simulink model "ControlePD_ind2015"  (R2015a)
settings: Solver=ode3  SolverMode=SingleTasking  StartTime=0.0  StopTime=10.0  FixedStep=Ts
values from neighbouring files (symbols this model uses):
  Beff = 50    [Ex4.m]
  Jeff = 2.2    [Ex4.m]
  K = 17.7    [Ex4.m]
  Kd = (2*qsi*wn*Jeff - Beff)/K    (= -0.338983050847)    [Ex4.m]
  Kp = (wn^2*Jeff)/K    (= 12.4293785311)    [Ex4.m]
  N = 10    [Ex4.m]
  r = 1    [Ex4.m]
  SP_theta = [60;-110;20;20;20]    [Ex4.m]
(part 1 of 3)
settings Model: CovMetricSettings=dwe  CovHtmlReporting=off  covSaveCumulativeToWorkspaceVar=off  CovSaveSingleToWorkspaceVar=off  CovExternalEMLEnable=on  Creator=Karoline  LastModifiedBy=lunet
settings DataIOCC: LimitDataPoints=off  SaveFormat=Dataset
settings DebuggingCC: SFUnexpectedBacktrackingDiag=error  SFNoUnconditionalDefaultTransitionDiag=error
settings HardwareCC: ProdBitPerPointer=64  ProdLargestAtomicFloat=Float  ProdIntDivRoundTo=Zero  ProdEndianess=LittleEndian  ProdHWDeviceType=Specified
settings ModelReferenceCC: PropagateSignalLabelsOutOfModel=on
settings GRTTargetCC: TargetLangStandard=C99 (ISO)

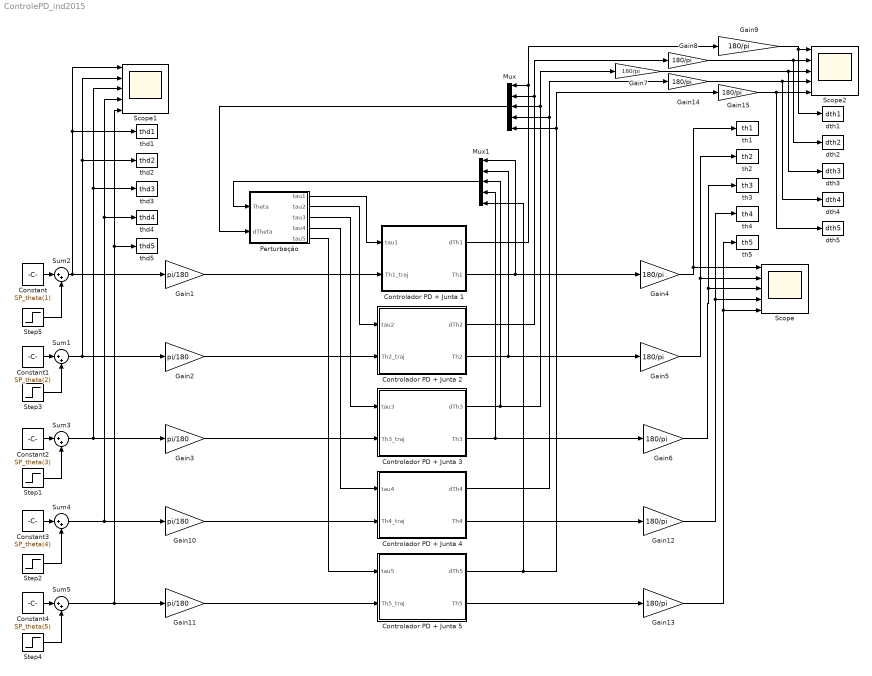
== system ControlePD_ind2015 ==
  Constant : Constant  Value=SP_theta(1)
  Constant1 : Constant  Value=SP_theta(2)
  Constant2 : Constant  Value=SP_theta(3)
  Constant3 : Constant  Value=SP_theta(4)
  Constant4 : Constant  Value=SP_theta(5)
  Controlador PD + Junta 1 : Subsystem
  Controlador PD + Junta 2 : Subsystem
  Controlador PD + Junta 3 : Subsystem
  Controlador PD + Junta 4 : Subsystem
  Controlador PD + Junta 5 : Subsystem
  Gain{1..3,10..11} (5 alike) : Gain  Gain=pi/180
  Gain{4..9,12..15} (10 alike) : Gain  Gain=180/pi
  Mux : Mux  Inputs=5
  Mux1 : Mux  Inputs=5
  Perturbação : Subsystem
  Scope : Scope  NumInputPorts=5
      settings: TimeRange=auto  MaxDataPoints=5000  SaveToWorkspace=off  SaveName=ScopeData  YMin=-133.87767~-5~-5~-5~-5  YMax=81.54196~5~5~5~5  SampleTime=-1
  Scope1 : Scope  NumInputPorts=5
      settings: TimeRange=auto  MaxDataPoints=5000  SaveToWorkspace=off  YMin=-131.25~-5~-5~-5~-5  YMax=81.25~5~5~5~5  SampleTime=-1
  Scope2 : Scope  NumInputPorts=5
      settings: TimeRange=auto  MaxDataPoints=5000  SaveToWorkspace=off  SaveName=ScopeData5  YMin=-33.93434~-5~-5~-5~-5  YMax=205.40908~5~5~5~5  SampleTime=-1
  Step{1..2,4..5} (4 alike) : Step  Time=0  After=0  SampleTime=0
  Step3 : Step  Time=3  After=60  SampleTime=0
  Sum{1..5} (5 alike) : Sum  Inputs=|++
  dth1 : ToWorkspace  VariableName=dth1  SampleTime=-1
  dth2 : ToWorkspace  VariableName=dth2  SampleTime=-1
  dth3 : ToWorkspace  VariableName=dth3  SampleTime=-1
  dth4 : ToWorkspace  VariableName=dth4  SampleTime=-1
  dth5 : ToWorkspace  VariableName=dth5  SampleTime=-1
  th1 : ToWorkspace  VariableName=th1  SampleTime=-1
  th2 : ToWorkspace  VariableName=th2  SampleTime=-1
  th3 : ToWorkspace  VariableName=th3  SampleTime=-1
  th4 : ToWorkspace  VariableName=th4  SampleTime=-1
  th5 : ToWorkspace  VariableName=th5  SampleTime=-1
  "thd1 " : ToWorkspace  VariableName=thd1  SampleTime=-1
  "thd2 " : ToWorkspace  VariableName=thd2  SampleTime=-1
  thd3 : ToWorkspace  VariableName=thd3  SampleTime=-1
  thd4 : ToWorkspace  VariableName=thd4  SampleTime=-1
  thd5 : ToWorkspace  VariableName=thd5  SampleTime=-1
  wires:
  Perturbação/1(tau1) -> Controlador PD + Junta 1/1(tau1)
  Mux/1 -> Perturbação/2(dTheta)
  Mux1/1 -> Perturbação/1(Theta)
  Step3/1 -> Sum1/2
  Sum1/1 -> Scope1/2, "thd2 "/1, Gain2/1
  Constant1/1 -> Sum1/1
  Gain1/1 -> Controlador PD + Junta 1/2(Th1_traj)
  Gain2/1 -> Controlador PD + Junta 2/2(Th2_traj)
  Gain3/1 -> Controlador PD + Junta 3/2(Th3_traj)
  Gain4/1 -> th1/1, Scope/1
  Gain5/1 -> th2/1, Scope/2
  Gain6/1 -> th3/1, Scope/3
  Controlador PD + Junta 1/1("dTh1 ") -> Mux/1, Gain9/1
  Controlador PD + Junta 2/1("dTh2 ") -> Mux/2, Gain8/1
  Controlador PD + Junta 3/1("dTh3 ") -> Mux1/3, Mux/3, Gain7/1
  Controlador PD + Junta 1/2(Th1) -> Mux1/1, Gain4/1
  Controlador PD + Junta 2/2(Th2) -> Mux1/2, Gain5/1
  Controlador PD + Junta 3/2(Th3) -> Mux1/4, Gain6/1
  Perturbação/2(tau2) -> Controlador PD + Junta 2/1(tau2)
  Perturbação/3(tau3) -> Controlador PD + Junta 3/1(tau3)
  Gain7/1 -> dth3/1, Scope2/3
  Gain8/1 -> dth2/1, Scope2/2
  Gain9/1 -> dth1/1, Scope2/1
  Gain10/1 -> Controlador PD + Junta 4/2(Th4_traj)
  Gain11/1 -> Controlador PD + Junta 5/2(Th5_traj)
  Constant/1 -> Sum2/1
  Constant2/1 -> Sum3/1
  Constant3/1 -> Sum4/1
  Constant4/1 -> Sum5/1
  Step1/1 -> Sum3/2
  Step2/1 -> Sum4/2
  Step4/1 -> Sum5/2
  Sum5/1 -> thd5/1, Scope1/5, Gain11/1
  Sum3/1 -> Gain3/1, Scope1/3, thd3/1
  Step5/1 -> Sum2/2
  Sum2/1 -> Scope1/1, "thd1 "/1, Gain1/1
  Sum4/1 -> thd4/1, Scope1/4, Gain10/1
  Controlador PD + Junta 4/2(Th4) -> Gain12/1
  Controlador PD + Junta 5/2(Th5) -> Gain13/1
  Gain12/1 -> Scope/4, th4/1
  Gain13/1 -> Scope/5, th5/1
  Gain14/1 -> dth4/1, Scope2/4
  Controlador PD + Junta 4/1("dTh4 ") -> Mux/4, Gain14/1
  Gain15/1 -> dth5/1, Scope2/5
  Controlador PD + Junta 5/1("dTh5 ") -> Mux1/5, Mux/5, Gain15/1
  Perturbação/4(tau4) -> Controlador PD + Junta 4/1(tau4)
  Perturbação/5(tau5) -> Controlador PD + Junta 5/1(tau5)

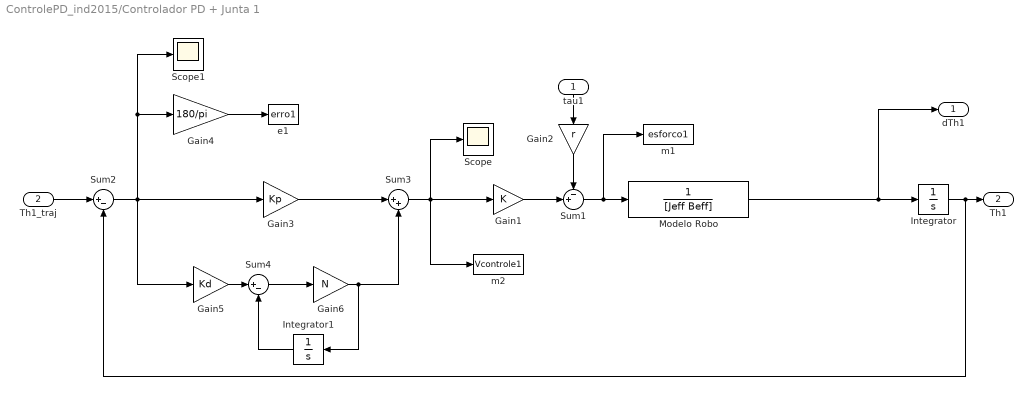
== system ControlePD_ind2015/Controlador PD + Junta 1 ==
  tau1 : Inport
  Th1_traj : Inport  Port=2
  Gain1 : Gain  Gain=K
  Gain2 : Gain  Gain=r
  Gain3 : Gain  Gain=Kp
  Gain4 : Gain  Gain=180/pi
  Gain5 : Gain  Gain=Kd
  Gain6 : Gain  Gain=N
  Integrator : Integrator  InitialCondition=SP_theta(1)*pi/180
  Integrator1 : Integrator
  Modelo Robo : TransferFcn  Denominator=[Jeff Beff]
  Scope : Scope
      settings: TimeRange=auto  MaxDataPoints=5000  SaveToWorkspace=off  YMin=-4.89691  YMax=11.84583  SampleTime=-1
  Scope1 : Scope
      settings: TimeRange=auto  MaxDataPoints=5000  SaveToWorkspace=off  SaveName=ScopeData6  YMin=-0.42473  YMax=1.21038  SampleTime=-1
  Sum1 : Sum  Inputs=-+|
  Sum2 : Sum  Inputs=|+-
  Sum3 : Sum  Inputs=|++
  Sum4 : Sum  Inputs=|+-
  e1 : ToWorkspace  VariableName=erro1  SampleTime=-1
  m1 : ToWorkspace  VariableName=esforco1  SampleTime=-1
  m2 : ToWorkspace  VariableName=Vcontrole1  SampleTime=-1
  "dTh1 " : Outport
  Th1 : Outport  Port=2
  wires:
  tau1/1 -> Gain2/1
  Gain1/1 -> Sum1/2
  Sum1/1 -> m1/1, Modelo Robo/1
  Integrator/1 -> Th1/1, Sum2/2
  Th1_traj/1 -> Sum2/1
  Gain2/1 -> Sum1/1
  Sum2/1 -> Gain5/1, Gain3/1, Scope1/1, Gain4/1
  Gain4/1 -> e1/1
  Gain3/1 -> Sum3/1
  Gain5/1 -> Sum4/1
  Sum4/1 -> Gain6/1
  Gain6/1 -> Sum3/2, Integrator1/1
  Integrator1/1 -> Sum4/2
  Sum3/1 -> m2/1, Scope/1, Gain1/1
  Modelo Robo/1 -> "dTh1 "/1, Integrator/1

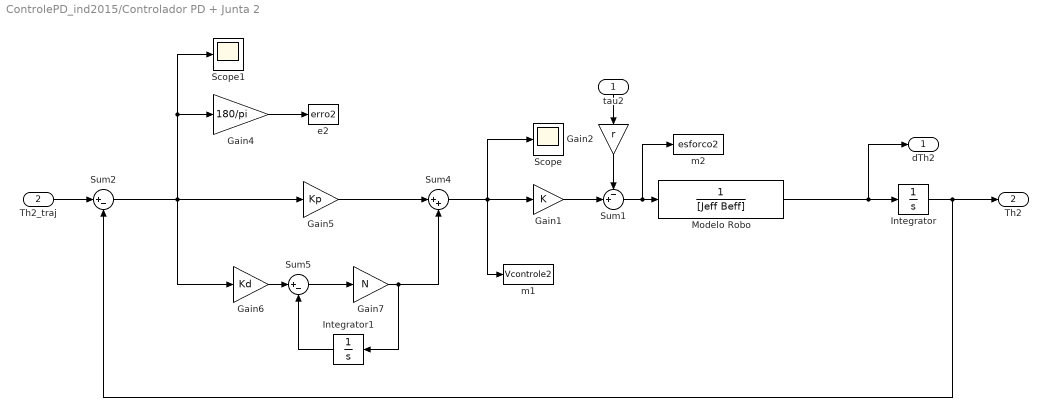
== system ControlePD_ind2015/Controlador PD + Junta 2 ==
  tau2 : Inport
  Th2_traj : Inport  Port=2
  Gain1 : Gain  Gain=K
  Gain2 : Gain  Gain=r
  Gain4 : Gain  Gain=180/pi
  Gain5 : Gain  Gain=Kp
  Gain6 : Gain  Gain=Kd
  Gain7 : Gain  Gain=N
  Integrator : Integrator  InitialCondition=SP_theta(2)*pi/180
  Integrator1 : Integrator
  "Modelo Robo " : TransferFcn  Denominator=[Jeff Beff]
  Scope : Scope
      settings: TimeRange=auto  MaxDataPoints=5000  SaveToWorkspace=off  SaveName=ScopeData2  YMin=-10  YMax=10  SampleTime=-1
  Scope1 : Scope
      settings: TimeRange=auto  MaxDataPoints=5000  SaveToWorkspace=off  SaveName=ScopeData5  YMin=-10  YMax=10  SampleTime=-1
  Sum1 : Sum  Inputs=-+|
  Sum2 : Sum  Inputs=|+-
  Sum4 : Sum  Inputs=|++
  Sum5 : Sum  Inputs=|+-
  e2 : ToWorkspace  VariableName=erro2  SampleTime=-1
  m1 : ToWorkspace  VariableName=Vcontrole2  SampleTime=-1
  m2 : ToWorkspace  VariableName=esforco2  SampleTime=-1
  "dTh2 " : Outport
  Th2 : Outport  Port=2
  wires:
  tau2/1 -> Gain2/1
  Gain1/1 -> Sum1/2
  Sum1/1 -> m2/1, "Modelo Robo "/1
  Integrator/1 -> Th2/1, Sum2/2
  Th2_traj/1 -> Sum2/1
  Gain2/1 -> Sum1/1
  Gain4/1 -> e2/1
  Gain5/1 -> Sum4/1
  Sum2/1 -> Scope1/1, Gain4/1, Gain6/1, Gain5/1
  Integrator1/1 -> Sum5/2
  Sum5/1 -> Gain7/1
  Gain6/1 -> Sum5/1
  Gain7/1 -> Sum4/2, Integrator1/1
  Sum4/1 -> m1/1, Scope/1, Gain1/1
  "Modelo Robo "/1 -> "dTh2 "/1, Integrator/1

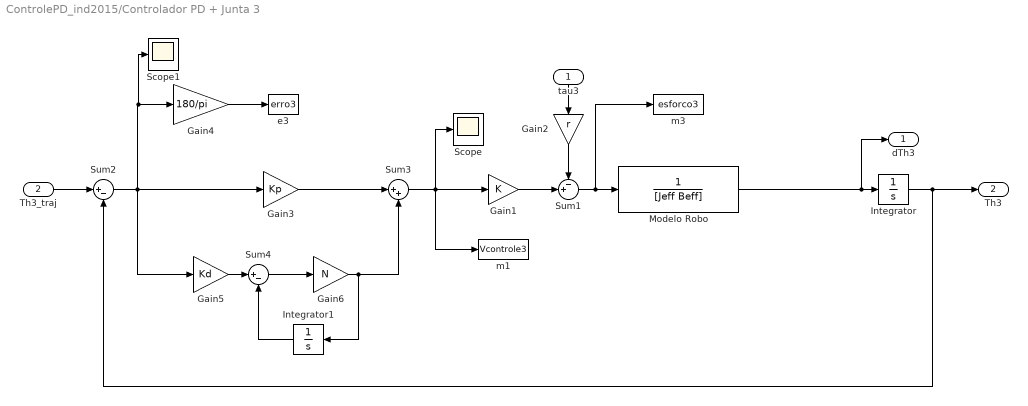
== system ControlePD_ind2015/Controlador PD + Junta 3 ==
  tau3 : Inport
  Th3_traj : Inport  Port=2
  Gain1 : Gain  Gain=K
  Gain2 : Gain  Gain=r
  Gain3 : Gain  Gain=Kp
  Gain4 : Gain  Gain=180/pi
  Gain5 : Gain  Gain=Kd
  Gain6 : Gain  Gain=N
  Integrator : Integrator  InitialCondition=SP_theta(3)*pi/180
  Integrator1 : Integrator
  Modelo Robo : TransferFcn  Denominator=[Jeff Beff]
  Scope : Scope
      settings: TimeRange=auto  MaxDataPoints=5000  SaveToWorkspace=off  SaveName=ScopeData3  YMin=-10  YMax=10  SampleTime=-1
  Scope1 : Scope
      settings: TimeRange=auto  MaxDataPoints=5000  SaveToWorkspace=off  SaveName=ScopeData4  YMin=-10  YMax=10  SampleTime=-1
  Sum1 : Sum  Inputs=-+|
  Sum2 : Sum  Inputs=|+-
  Sum3 : Sum  Inputs=|++
  Sum4 : Sum  Inputs=|+-
  e3 : ToWorkspace  VariableName=erro3  SampleTime=-1
  m1 : ToWorkspace  VariableName=Vcontrole3  SampleTime=-1
  m3 : ToWorkspace  VariableName=esforco3  SampleTime=-1
  "dTh3 " : Outport
  Th3 : Outport  Port=2
  wires:
  tau3/1 -> Gain2/1
  Gain1/1 -> Sum1/2
  Sum1/1 -> m3/1, Modelo Robo/1
  Integrator/1 -> Th3/1, Sum2/2
  Th3_traj/1 -> Sum2/1
  Gain2/1 -> Sum1/1
  Gain4/1 -> e3/1
  Gain3/1 -> Sum3/1
  Sum2/1 -> Scope1/1, Gain4/1, Gain5/1, Gain3/1
  Integrator1/1 -> Sum4/2
  Sum4/1 -> Gain6/1
  Gain5/1 -> Sum4/1
  Gain6/1 -> Sum3/2, Integrator1/1
  Sum3/1 -> m1/1, Scope/1, Gain1/1
  Modelo Robo/1 -> Integrator/1, "dTh3 "/1

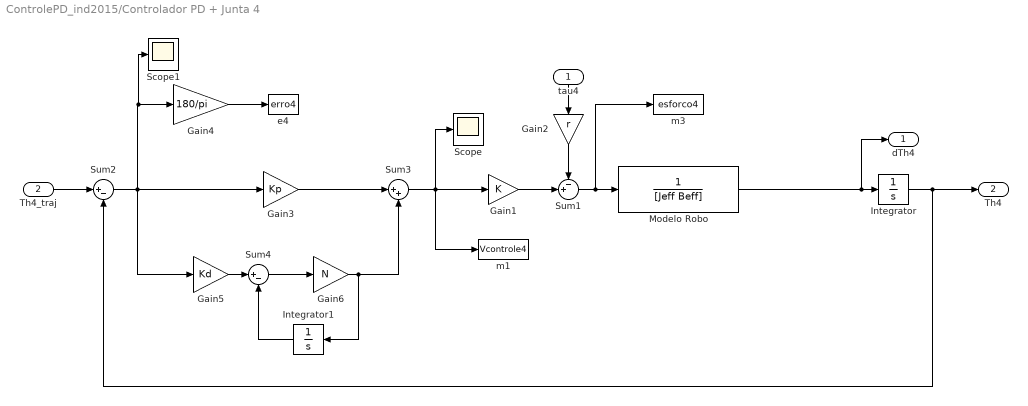
== system ControlePD_ind2015/Controlador PD + Junta 4 ==
  tau4 : Inport
  Th4_traj : Inport  Port=2
  Gain1 : Gain  Gain=K
  Gain2 : Gain  Gain=r
  Gain3 : Gain  Gain=Kp
  Gain4 : Gain  Gain=180/pi
  Gain5 : Gain  Gain=Kd
  Gain6 : Gain  Gain=N
  Integrator : Integrator  InitialCondition=SP_theta(4)*pi/180
  Integrator1 : Integrator
  Modelo Robo : TransferFcn  Denominator=[Jeff Beff]
  Scope : Scope
      settings: TimeRange=auto  MaxDataPoints=5000  SaveToWorkspace=off  SaveName=ScopeData3  YMin=-10  YMax=10  SampleTime=-1
  Scope1 : Scope
      settings: TimeRange=auto  MaxDataPoints=5000  SaveToWorkspace=off  SaveName=ScopeData4  YMin=-10  YMax=10  SampleTime=-1
  Sum1 : Sum  Inputs=-+|
  Sum2 : Sum  Inputs=|+-
  Sum3 : Sum  Inputs=|++
  Sum4 : Sum  Inputs=|+-
  e4 : ToWorkspace  VariableName=erro4  SampleTime=-1
  m1 : ToWorkspace  VariableName=Vcontrole4  SampleTime=-1
  m3 : ToWorkspace  VariableName=esforco4  SampleTime=-1
  "dTh4 " : Outport
  Th4 : Outport  Port=2
  wires:
  tau4/1 -> Gain2/1
  Gain1/1 -> Sum1/2
  Sum1/1 -> m3/1, Modelo Robo/1
  Integrator/1 -> Th4/1, Sum2/2
  Th4_traj/1 -> Sum2/1
  Gain2/1 -> Sum1/1
  Gain4/1 -> e4/1
  Gain3/1 -> Sum3/1
  Sum2/1 -> Scope1/1, Gain4/1, Gain5/1, Gain3/1
  Integrator1/1 -> Sum4/2
  Sum4/1 -> Gain6/1
  Gain5/1 -> Sum4/1
  Gain6/1 -> Sum3/2, Integrator1/1
  Sum3/1 -> m1/1, Scope/1, Gain1/1
  Modelo Robo/1 -> Integrator/1, "dTh4 "/1

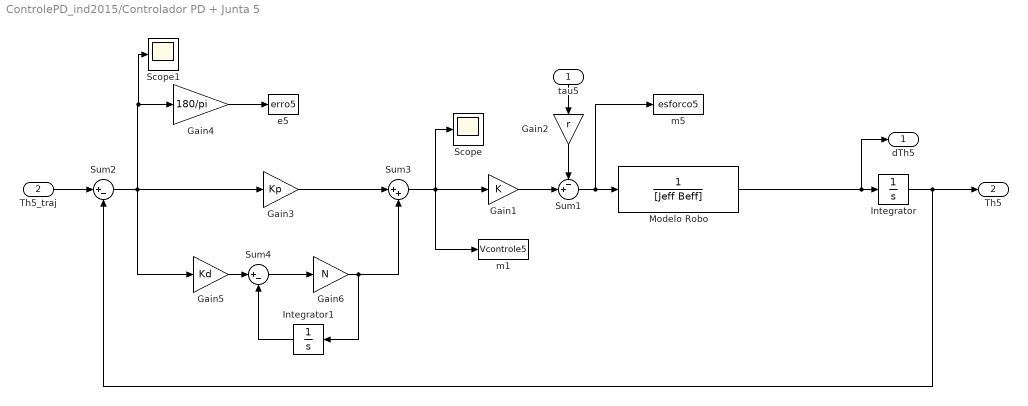
== system ControlePD_ind2015/Controlador PD + Junta 5 ==
  tau5 : Inport
  Th5_traj : Inport  Port=2
  Gain1 : Gain  Gain=K
  Gain2 : Gain  Gain=r
  Gain3 : Gain  Gain=Kp
  Gain4 : Gain  Gain=180/pi
  Gain5 : Gain  Gain=Kd
  Gain6 : Gain  Gain=N
  Integrator : Integrator  InitialCondition=SP_theta(5)*pi/180
  Integrator1 : Integrator
  Modelo Robo : TransferFcn  Denominator=[Jeff Beff]
  Scope : Scope
      settings: TimeRange=auto  MaxDataPoints=5000  SaveToWorkspace=off  SaveName=ScopeData3  YMin=-10  YMax=10  SampleTime=-1
  Scope1 : Scope
      settings: TimeRange=auto  MaxDataPoints=5000  SaveToWorkspace=off  SaveName=ScopeData4  YMin=-10  YMax=10  SampleTime=-1
  Sum1 : Sum  Inputs=-+|
  Sum2 : Sum  Inputs=|+-
  Sum3 : Sum  Inputs=|++
  Sum4 : Sum  Inputs=|+-
  e5 : ToWorkspace  VariableName=erro5  SampleTime=-1
  m1 : ToWorkspace  VariableName=Vcontrole5  SampleTime=-1
  m5 : ToWorkspace  VariableName=esforco5  SampleTime=-1
  "dTh5 " : Outport
  Th5 : Outport  Port=2
  wires:
  tau5/1 -> Gain2/1
  Gain1/1 -> Sum1/2
  Sum1/1 -> m5/1, Modelo Robo/1
  Integrator/1 -> Th5/1, Sum2/2
  Th5_traj/1 -> Sum2/1
  Gain2/1 -> Sum1/1
  Gain4/1 -> e5/1
  Gain3/1 -> Sum3/1
  Sum2/1 -> Scope1/1, Gain4/1, Gain5/1, Gain3/1
  Integrator1/1 -> Sum4/2
  Sum4/1 -> Gain6/1
  Gain5/1 -> Sum4/1
  Gain6/1 -> Sum3/2, Integrator1/1
  Sum3/1 -> m1/1, Scope/1, Gain1/1
  Modelo Robo/1 -> Integrator/1, "dTh5 "/1

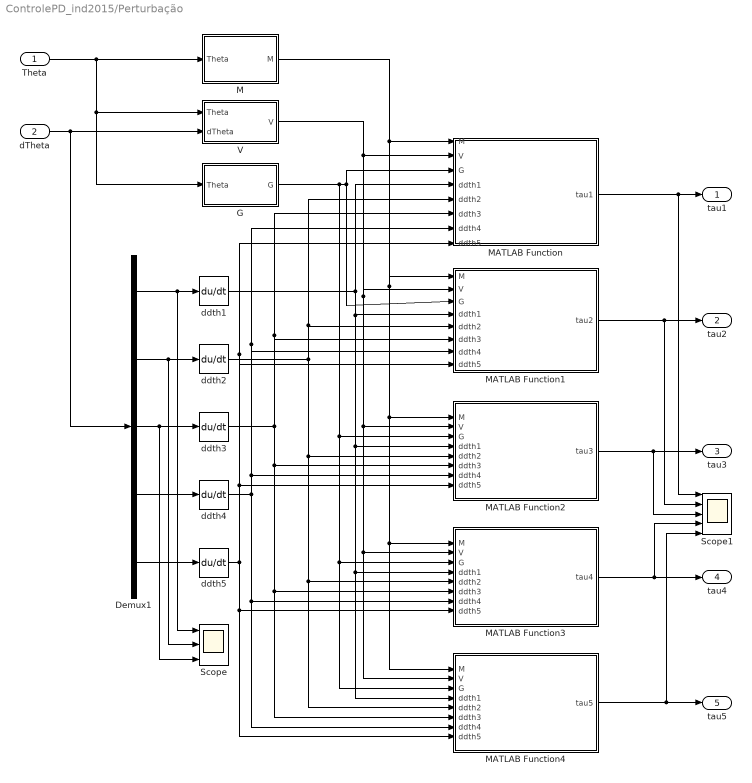
== system ControlePD_ind2015/Perturbação ==
  Theta : Inport
  dTheta : Inport  Port=2
  Demux1 : Demux  Outputs=5
  G : Subsystem
  M : Subsystem
  MATLAB Function : MATLAB Function  TreatAsAtomicUnit=on
      settings: PermitHierarchicalResolution=ParametersOnly
  MATLAB Function1 : MATLAB Function  TreatAsAtomicUnit=on
      settings: PermitHierarchicalResolution=ParametersOnly
  MATLAB Function2 : MATLAB Function  TreatAsAtomicUnit=on
      settings: PermitHierarchicalResolution=ParametersOnly
  MATLAB Function3 : MATLAB Function  TreatAsAtomicUnit=on
      settings: PermitHierarchicalResolution=ParametersOnly
  MATLAB Function4 : MATLAB Function  TreatAsAtomicUnit=on
      settings: PermitHierarchicalResolution=ParametersOnly
  Scope : Scope  NumInputPorts=3
      settings: TimeRange=auto  MaxDataPoints=5000  SaveToWorkspace=off  SaveName=ScopeData6  YMin=-10~-5~-5  YMax=10~5~5  SampleTime=-1
  Scope1 : Scope  NumInputPorts=5
      settings: TimeRange=auto  MaxDataPoints=5000  SaveToWorkspace=off  SaveName=ScopeData7  YMin=-10~-5~-5~-5~-5  YMax=10~5~5~5~5  SampleTime=-1
  V : Subsystem
  ddth{1..5} (5 alike) : Derivative
  tau1 : Outport
  tau2 : Outport  Port=2
  tau3 : Outport  Port=3
  tau4 : Outport  Port=4
  tau5 : Outport  Port=5
  wires:
  dTheta/1 -> Demux1/1, V/2(dTheta)
  G/1(G) -> MATLAB Function1/3(G), MATLAB Function/3(G), MATLAB Function4/3(G), MATLAB Function3/3(G), MATLAB Function2/3(G)
  V/1(V) -> MATLAB Function1/2(V), MATLAB Function4/2(V), MATLAB Function3/2(V), MATLAB Function2/2(V), MATLAB Function/2(V)
  Theta/1 -> M/1(Theta), G/1(Theta), V/1(Theta)
  Demux1/1 -> Scope/1, ddth1/1
  Demux1/2 -> Scope/2, ddth2/1
  Demux1/3 -> Scope/3, ddth3/1
  MATLAB Function/1(tau1) -> tau1/1, Scope1/1
  MATLAB Function1/1(tau2) -> tau2/1, Scope1/2
  MATLAB Function2/1(tau3) -> Scope1/3, tau3/1
  Demux1/4 -> ddth4/1
  Demux1/5 -> ddth5/1
  M/1(M) -> MATLAB Function4/1(M), MATLAB Function3/1(M), MATLAB Function2/1(M), MATLAB Function1/1(M), MATLAB Function/1(M)
  ddth1/1 -> MATLAB Function4/4(ddth1), MATLAB Function3/4(ddth1), MATLAB Function2/4(ddth1), MATLAB Function1/4(ddth1), MATLAB Function/4(ddth1)
  ddth2/1 -> MATLAB Function4/5(ddth2), MATLAB Function3/5(ddth2), MATLAB Function2/5(ddth2), MATLAB Function1/5(ddth2), MATLAB Function/5(ddth2)
  ddth3/1 -> MATLAB Function1/6(ddth3), MATLAB Function/6(ddth3), MATLAB Function4/6(ddth3), MATLAB Function3/6(ddth3), MATLAB Function2/6(ddth3)
  ddth4/1 -> MATLAB Function2/7(ddth4), MATLAB Function1/7(ddth4), MATLAB Function/7(ddth4), MATLAB Function4/7(ddth4), MATLAB Function3/7(ddth4)
  ddth5/1 -> MATLAB Function2/8(ddth5), MATLAB Function1/8(ddth5), MATLAB Function/8(ddth5), MATLAB Function4/8(ddth5), MATLAB Function3/8(ddth5)
  MATLAB Function3/1(tau4) -> Scope1/4, tau4/1
  MATLAB Function4/1(tau5) -> Scope1/5, tau5/1

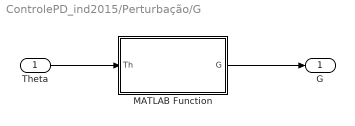
== system ControlePD_ind2015/Perturbação/G ==
  Theta : Inport
  MATLAB Function : MATLAB Function  TreatAsAtomicUnit=on
      settings: PermitHierarchicalResolution=ParametersOnly
  G : Outport
  wires:
  Theta/1 -> MATLAB Function/1(Th)
  MATLAB Function/1(G) -> G/1

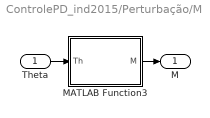
== system ControlePD_ind2015/Perturbação/M ==
  Theta : Inport
  MATLAB Function3 : MATLAB Function  TreatAsAtomicUnit=on
      settings: PermitHierarchicalResolution=ParametersOnly
  M : Outport
  wires:
  Theta/1 -> MATLAB Function3/1(Th)
  MATLAB Function3/1(M) -> M/1

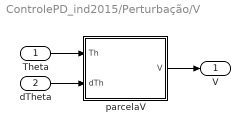
== system ControlePD_ind2015/Perturbação/V ==
  Theta : Inport
  dTheta : Inport  Port=2
  parcelaV : MATLAB Function  TreatAsAtomicUnit=on
      settings: PermitHierarchicalResolution=ParametersOnly
  V : Outport
  wires:
  parcelaV/1(V) -> V/1
  Theta/1 -> parcelaV/1(Th)
  dTheta/1 -> parcelaV/2(dTh)

== matlab function ControlePD_ind2015/Perturbação/MATLAB Function3 ==
  data: M input; V input; tau4 output; G input; ddth1 input; ddth2 input; ddth3 input; ddth4 input; ddth5 input
function tau4  = calcul_dk4(M, V, G,ddth1,ddth2,ddth3,ddth4,ddth5)

ddth = [ddth1; ddth2; ddth3; ddth4; ddth5];

tau4 = M(4,:)*ddth + V(4,1) + G(4);

== matlab function ControlePD_ind2015/Perturbação/G/MATLAB Function ==
  data: Th input; G output
function G = calcul_G(Th)

th1 = Th(1);
th2 = Th(2);
th3 = Th(3);
th4 = Th(4);
th5 = Th(5);
g = 9.81;

G = [                                                                                                                                                                                                                                                                                               0;
 -g*((49*cos(th2)*sin(th3))/125 - cos(th2)/2 + (49*cos(th3)*sin(th2))/125 + (3*cos(th2)*cos(th5)*sin(th3))/40 + (3*cos(th3)*cos(th5)*sin(th2))/40 + (3*cos(th2)*cos(th3)*cos(th4)*sin(th5))/40 - (3*cos(th4)*sin(th2)*sin(th3)*sin(th5))/40);
                 -g*((49*cos(th2)*sin(th3))/125 + (49*cos(th3)*sin(th2))/125 + (3*cos(th2)*cos(th5)*sin(th3))/40 + (3*cos(th3)*cos(th5)*sin(th2))/40 + (3*cos(th2)*cos(th3)*cos(th4)*sin(th5))/40 - (3*cos(th4)*sin(th2)*sin(th3)*sin(th5))/40);
                                                                                                                                                                                                                                                (3*g*sin(th4)*sin(th5)*sin(th2 + th3))/40;
                                                                                       -g*((3*cos(th2)*cos(th3)*sin(th5))/40 - (3*sin(th2)*sin(th3)*sin(th5))/40 + (3*cos(th2)*cos(th4)*cos(th5)*sin(th3))/40 + (3*cos(th3)*cos(th4)*cos(th5)*sin(th2))/40)];

== matlab function ControlePD_ind2015/Perturbação/MATLAB Function1 ==
  data: M input; V input; tau2 output; G input; ddth1 input; ddth2 input; ddth3 input; ddth4 input; ddth5 input
function tau2  = calcul_dk2(M,V,G,ddth1,ddth2,ddth3,ddth4,ddth5)

ddth = [ddth1; ddth2; ddth3; ddth4; ddth5];

tau2 = M(2,:)*ddth + V(2,1) + G(2);

== matlab function ControlePD_ind2015/Perturbação/MATLAB Function ==
  data: M input; V input; tau1 output; G input; ddth1 input; ddth2 input; ddth3 input; ddth4 input; ddth5 input
function tau1  = calcul_dk1(M,V,G,ddth1,ddth2,ddth3,ddth4,ddth5)

ddth = [ddth1; ddth2; ddth3; ddth4; ddth5];

tau1 = M(1,:)*ddth + V(1,1) + G(1);

== matlab function ControlePD_ind2015/Perturbação/MATLAB Function2 ==
  data: M input; V input; tau3 output; G input; ddth1 input; ddth2 input; ddth3 input; ddth4 input; ddth5 input
function tau3  = calcul_dk3(M, V, G,ddth1,ddth2,ddth3,ddth4,ddth5)

ddth = [ddth1; ddth2; ddth3; ddth4; ddth5];

tau3 = M(3,:)*ddth + V(3,1) + G(3);

== matlab function ControlePD_ind2015/Perturbação/M/MATLAB Function3 ==
  data: Th input; M output
function M = calcul_M(Th)

th1 = Th(1);
th2 = Th(2);
th3 = Th(3);
th4 = Th(4);
th5 = Th(5);

M = [ (87*cos(th2)^2*cos(th5))/2500 + (87*cos(th3)^2*cos(th5))/2500 - (33*cos(th2)^2*sin(th3))/50 + (53231*cos(th2)^2)/62500 + (8453*cos(th3)^2)/31250 - (9*cos(th5)^2)/3200 - (8453*cos(th2)^2*cos(th3)^2)/15625 - (217*cos(th2)^2*cos(th4)^2)/80000 + (9*cos(th2)^2*cos(th5)^2)/3200 - (217*cos(th3)^2*cos(th4)^2)/80000 + (9*cos(th3)^2*cos(th5)^2)/3200 - (87*cos(th2)^2*cos(th3)^2*cos(th5))/1250 - (33*cos(th2)*cos(th3)*sin(th2))/50 + (217*cos(th2)^2*cos(th3)^2*cos(th4)^2)/40000 - (9*cos(th2)^2*cos(th3)^2*cos(th5)^2)/1600 + (9*cos(th2)^2*cos(th4)^2*cos(th5)^2)/3200 + (9*cos(th3)^2*cos(th4)^2*cos(th5)^2)/3200 - (3*cos(th2)^2*cos(th5)*sin(th3))/80 - (9*cos(th2)^2*cos(th3)^2*cos(th4)^2*cos(th5)^2)/1600 - (3*cos(th2)*cos(th3)*cos(th5)*sin(th2))/80 + (8453*cos(th2)*cos(th3)*sin(th2)*sin(th3))/15625 - (87*cos(th2)*cos(th4)*sin(th2)*sin(th5))/2500 - (87*cos(th3)*cos(th4)*sin(th3)*sin(th5))/2500 - (3*cos(th2)^2*cos(th3)*cos(th4)*sin(th5))/80 + (3*cos(th2)*cos(th4)*sin(th2)*sin(th3)*sin(th5))/80 - (217*cos(th2)*cos(th3)*cos(th4)^2*sin(th2)*sin(th3))/40000 + (9*cos(th2)*cos(th3)*cos(th5)^2*sin(th2)*sin(th3))/1600 + (87*cos(th2)*cos(th3)^2*cos(th4)*sin(th2)*sin(th5))/1250 + (87*cos(th2)^2*cos(th3)*cos(th4)*sin(th3)*sin(th5))/1250 + (87*cos(th2)*cos(th3)*cos(th5)*sin(th2)*sin(th3))/1250 - (9*cos(th2)*cos(th4)*cos(th5)*sin(th2)*sin(th5))/1600 - (9*cos(th3)*cos(th4)*cos(th5)*sin(th3)*sin(th5))/1600 + (9*cos(th2)*cos(th3)*cos(th4)^2*cos(th5)^2*sin(th2)*sin(th3))/1600 + (9*cos(th2)*cos(th3)^2*cos(th4)*cos(th5)*sin(th2)*sin(th5))/800 + (9*cos(th2)^2*cos(th3)*cos(th4)*cos(th5)*sin(th3)*sin(th5))/800 + 3793/80000, -(sin(th4)*(1500*sin(th2)*sin(th5) - 217*cos(th2)*cos(th4)*sin(th3) - 217*cos(th3)*cos(th4)*sin(th2) + 1392*cos(th2)*cos(th3)*sin(th5) - 1392*sin(th2)*sin(th3)*sin(th5) + 225*cos(th2)*cos(th3)*cos(th5)*sin(th5) - 225*cos(th5)*sin(th2)*sin(th3)*sin(th5) + 225*cos(th2)*cos(th4)*cos(th5)^2*sin(th3) + 225*cos(th3)*cos(th4)*cos(th5)^2*sin(th2)))/80000, (sin(th4)*(217*cos(th2)*cos(th4)*sin(th3) + 217*cos(th3)*cos(th4)*sin(th2) - 1392*cos(th2)*cos(th3)*sin(th5) + 1392*sin(th2)*sin(th3)*sin(th5) - 225*cos(th2)*cos(th3)*cos(th5)*sin(th5) + 225*cos(th5)*sin(th2)*sin(th3)*sin(th5) - 225*cos(th2)*cos(th4)*cos(th5)^2*sin(th3) - 225*cos(th3)*cos(th4)*cos(th5)^2*sin(th2)))/80000, (489*cos(th2)*cos(th3))/80000 - (489*sin(th2)*sin(th3))/80000 - (3*cos(th2)*cos(th4)*sin(th5))/160 - (9*cos(th2)*cos(th3)*cos(th5)^2)/3200 + (9*cos(th5)^2*sin(th2)*sin(th3))/3200 + (87*cos(th2)*cos(th4)*sin(th3)*sin(th5))/5000 + (87*cos(th3)*cos(th4)*sin(th2)*sin(th5))/5000 + (9*cos(th2)*cos(th4)*cos(th5)*sin(th3)*sin(th5))/3200 + (9*cos(th3)*cos(th4)*cos(th5)*sin(th2)*sin(th5))/3200, (sin(th4)*(353*cos(th2)*sin(th3) + 353*cos(th3)*sin(th2) - 1500*cos(th2)*cos(th5) + 1392*cos(th2)*cos(th5)*sin(th3) + 1392*cos(th3)*cos(th5)*sin(th2)))/80000;
                                                                                                                                                                                                                                                                                                                                                                                                                                                                                                                                                                                                                                                                                                                                                                                                                                                                                                                                                                                                                                                                                                                                                                                                                                                                                                                                                                                                                                                                                                                                                                                            -(sin(th4)*(1500*sin(th2)*sin(th5) - 217*cos(th2)*cos(th4)*sin(th3) - 217*cos(th3)*cos(th4)*sin(th2) + 1392*cos(th2)*cos(th3)*sin(th5) - 1392*sin(th2)*sin(th3)*sin(th5) + 225*cos(th2)*cos(th3)*cos(th5)*sin(th5) - 225*cos(th5)*sin(th2)*sin(th3)*sin(th5) + 225*cos(th2)*cos(th4)*cos(th5)^2*sin(th3) + 225*cos(th3)*cos(th4)*cos(th5)^2*sin(th2)))/80000,                                                                                                                                                                                                                       (87*cos(th5))/2500 - (33*sin(th3))/50 - (3*cos(th5)*sin(th3))/80 + (217*cos(th4)^2)/80000 + (9*cos(th5)^2)/3200 - (9*cos(th4)^2*cos(th5)^2)/3200 - (3*cos(th3)*cos(th4)*sin(th5))/80 + 54781/62500,                                                                                                                                                                                   (87*cos(th5))/2500 - (33*sin(th3))/100 - (3*cos(th5)*sin(th3))/160 + (217*cos(th4)^2)/80000 + (9*cos(th5)^2)/3200 - (9*cos(th4)^2*cos(th5)^2)/3200 - (3*cos(th3)*cos(th4)*sin(th5))/160 + 72749/250000,                                                                                                                                                                                                                                                                                                                                                                                                                     -(3*sin(th4)*sin(th5)*(75*cos(th5) - 500*sin(th3) + 464))/80000,                                                          (353*cos(th4))/80000 - (3*cos(th3)*sin(th5))/160 + (87*cos(th4)*cos(th5))/5000 - (3*cos(th4)*cos(th5)*sin(th3))/160;
                                                                                                                                                                                                                                                                                                                                                                                                                                                                                                                                                                                                                                                                                                                                                                                                                                                                                                                                                                                                                                                                                                                                                                                                                                                                                                                                                                                                                                                                                                                                                                                                                            (sin(th4)*(217*cos(th2)*cos(th4)*sin(th3) + 217*cos(th3)*cos(th4)*sin(th2) - 1392*cos(th2)*cos(th3)*sin(th5) + 1392*sin(th2)*sin(th3)*sin(th5) - 225*cos(th2)*cos(th3)*cos(th5)*sin(th5) + 225*cos(th5)*sin(th2)*sin(th3)*sin(th5) - 225*cos(th2)*cos(th4)*cos(th5)^2*sin(th3) - 225*cos(th3)*cos(th4)*cos(th5)^2*sin(th2)))/80000,                                                                                                                                                                                                                   (87*cos(th5))/2500 - (33*sin(th3))/100 - (3*cos(th5)*sin(th3))/160 + (217*cos(th4)^2)/80000 + (9*cos(th5)^2)/3200 - (9*cos(th4)^2*cos(th5)^2)/3200 - (3*cos(th3)*cos(th4)*sin(th5))/160 + 72749/250000,                                                                                                                                                                                                                                                                                          (87*cos(th5))/2500 + (217*cos(th4)^2)/80000 + (9*cos(th5)^2)/3200 - (9*cos(th4)^2*cos(th5)^2)/3200 + 72749/250000,                                                                                                                                                                                                                                                                                                                                                                                                                                       -(3*sin(th4)*sin(th5)*(75*cos(th5) + 464))/80000,                                                                                                                                                         (cos(th4)*(1392*cos(th5) + 353))/80000;
                                                                                                                                                                                                                                                                                                                                                                                                                                                                                                                                                                                                                                                                                                                                                                                                                                                                                                                                                                                                                                                                                                                                                                                                                                                                                                                                                                                                                                                                                                                                                      (489*cos(th2)*cos(th3))/80000 - (489*sin(th2)*sin(th3))/80000 - (3*cos(th2)*cos(th4)*sin(th5))/160 - (9*cos(th2)*cos(th3)*cos(th5)^2)/3200 + (9*cos(th5)^2*sin(th2)*sin(th3))/3200 + (87*cos(th2)*cos(th4)*sin(th3)*sin(th5))/5000 + (87*cos(th3)*cos(th4)*sin(th2)*sin(th5))/5000 + (9*cos(th2)*cos(th4)*cos(th5)*sin(th3)*sin(th5))/3200 + (9*cos(th3)*cos(th4)*cos(th5)*sin(th2)*sin(th5))/3200,                                                                                                                                                                                                                                                                                                                                                                               -(3*sin(th4)*sin(th5)*(75*cos(th5) - 500*sin(th3) + 464))/80000,                                                                                                                                                                                                                                                                                                                                                                 -(3*sin(th4)*sin(th5)*(75*cos(th5) + 464))/80000,                                                                                                                                                                                                                                                                                                                                                                                                                                                              489/80000 - (9*cos(th5)^2)/3200,                                                                                                                                                                                                    0;
                                                                                                                                                                                                                                                                                                                                                                                                                                                                                                                                                                                                                                                                                                                                                                                                                                                                                                                                                                                                                                                                                                                                                                                                                                                                                                                                                                                                                                                                                                                                                                                                                                                                                                                                                                                                                                                 (sin(th4)*(353*cos(th2)*sin(th3) + 353*cos(th3)*sin(th2) - 1500*cos(th2)*cos(th5) + 1392*cos(th2)*cos(th5)*sin(th3) + 1392*cos(th3)*cos(th5)*sin(th2)))/80000,                                                                                                                                                                                                                                                                                                               (353*cos(th4))/80000 - (3*cos(th3)*sin(th5))/160 + (87*cos(th4)*cos(th5))/5000 - (3*cos(th4)*cos(th5)*sin(th3))/160,                                                                                                                                                                                                                                                                                                                                                                              (cos(th4)*(1392*cos(th5) + 353))/80000,                                                                                                                                                                                                                                                                                                                                                                                                                                                                                               0,                                                                                                                                                                                            353/80000];
